simulink model "sistemi_me_vonese_variabile"  (R2016b)
settings: Solver=VariableStepAuto  StartTime=0.0  StopTime=100  MaxStep=0.01  RelTol=1e-3
libraries: simulink x1
settings Model: Creator=aidbu  LastModifiedBy=aidbu

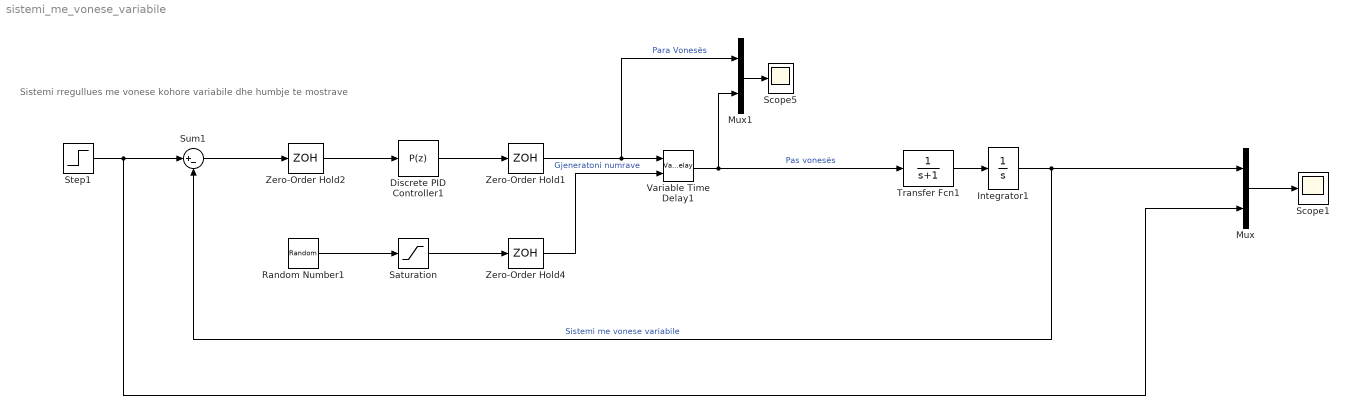
== system sistemi_me_vonese_variabile ==
  note: Sistemi rregullues me vonese kohore variabile dhe humbje te mostrave
  Discrete PID Controller1 : simulink/Continuous/PID Controller  Controller=P  TimeDomain=Discrete-time  SampleTime=0.1  IntegratorMethod=Forward Euler  FilterMethod=Forward Euler  Form=Parallel  UseFilter=on  ControllerParametersSource=internal  P=0.6159  I=0.3369  D=1.551  N=18.21  InitialConditionSource=internal  InitialConditionForIntegrator=0  InitialConditionForFilter=0  ExternalReset=none  LimitOutput=off  UpperSaturationLimit=inf  LowerSaturationLimit=-inf  LinearizeAsGain=off  AntiWindupMode=none  Kb=1  TrackingMode=off  Kt=1  PParamMin=[]  PParamMax=[]  IParamMin=[]  IParamMax=[]  DParamMin=[]  DParamMax=[]  NParamMin=[]  NParamMax=[]  KbParamMin=[]  KbParamMax=[]  KtParamMin=[]  KtParamMax=[]  POutMin=[]  POutMax=[]  IOutMin=[]  IOutMax=[]  DOutMin=[]  DOutMax=[]  NOutMin=[]  NOutMax=[]  KbOutMin=[]  KbOutMax=[]  KtOutMin=[]  KtOutMax=[]  IntegratorOutMin=[]  IntegratorOutMax=[]  FilterOutMin=[]  FilterOutMax=[]  SumOutMin=[]  SumOutMax=[]  SumI1OutMin=[]  SumI1OutMax=[]  SumI2OutMin=[]  SumI2OutMax=[]  SumI3OutMin=[]  SumI3OutMax=[]  SumDOutMin=[]  SumDOutMax=[]  SaturationOutMin=[]  SaturationOutMax=[]  IntegratorContinuousStateAttributes=''  IntegratorStateMustResolveToSignalObject=off  IntegratorRTWStateStorageClass=Auto  FilterContinuousStateAttributes=''  FilterStateMustResolveToSignalObject=off  FilterRTWStateStorageClass=Auto  DifferentiatorICPrevScaledInput=0  DifferentiatorOutMin=[]  DifferentiatorOutMax=[]
  Integrator1 : Integrator
  Mux : Mux  Inputs=2
  Mux1 : Mux  Inputs=2
  Random Number1 : RandomNumber  Mean=0.05  Variance=0.001  Seed=1  SampleTime=0.1
  Saturation : Saturate  UpperLimit=0.09  LowerLimit=0.01
  Scope1 : Scope
  Scope5 : Scope
  Step1 : Step  Time=0  SampleTime=0
  Sum1 : Sum  Inputs=|+-
  Transfer Fcn1 : TransferFcn  Denominator=[1 1]
  Variable Time Delay1 : VariableTransportDelay  MaximumDelay=0.1
  Zero-Order Hold1 : ZeroOrderHold  SampleTime=0.1
  Zero-Order Hold2 : ZeroOrderHold  SampleTime=5
  Zero-Order Hold4 : ZeroOrderHold  SampleTime=0.1
  wires:
  Step1/1 -> Mux/2, Sum1/1
  Sum1/1 -> Zero-Order Hold2/1
  Zero-Order Hold2/1 -> Discrete PID Controller1/1
  Discrete PID Controller1/1 -> Zero-Order Hold1/1
  Zero-Order Hold1/1 -> Mux1/1, Variable Time Delay1/1  "Para Vonesës"
  Transfer Fcn1/1 -> Integrator1/1
  Integrator1/1 -> Sum1/2, Mux/1  "Sistemi me vonese variabile"
  Variable Time Delay1/1 -> Mux1/2, Transfer Fcn1/1  "Pas vonesës"
  Random Number1/1 -> Saturation/1
  Mux1/1 -> Scope5/1
  Zero-Order Hold4/1 -> Variable Time Delay1/2  "Gjeneratoni numrave"
  Saturation/1 -> Zero-Order Hold4/1
  Mux/1 -> Scope1/1
